simulink model "upperLimb"  (R2017b)
settings: Solver=VariableStepAuto  StartTime=0.0  StopTime=10.0  RelTol=1e-3
settings Model: Creator=user  LastModifiedBy=user

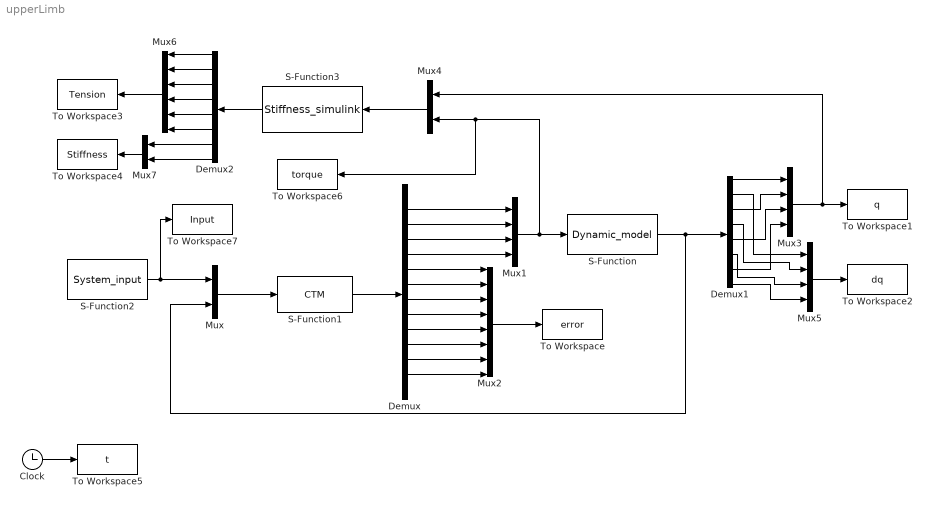
== system upperLimb ==
  Clock : Clock
  Demux : Demux  Outputs=12
  Demux1 : Demux  Outputs=8
  Demux2 : Demux  Outputs=8
  Mux : Mux  Inputs=2
  Mux1 : Mux
  Mux2 : Mux  Inputs=8
  Mux3 : Mux
  Mux4 : Mux  Inputs=2
  Mux5 : Mux
  Mux6 : Mux  Inputs=6
  Mux7 : Mux  Inputs=2
  S-Function : S-Function  FunctionName=Dynamic_model  SFunctionDeploymentMode=off  EnableBusSupport=off
  S-Function1 : S-Function  FunctionName=CTM  SFunctionDeploymentMode=off  EnableBusSupport=off
  S-Function2 : S-Function  FunctionName=System_input  SFunctionDeploymentMode=off  EnableBusSupport=off
  S-Function3 : S-Function  FunctionName=Stiffness_simulink  SFunctionDeploymentMode=off  EnableBusSupport=off
  To Workspace : ToWorkspace  VariableName=error  SaveFormat=Timeseries  SampleTime=-1
  To Workspace1 : ToWorkspace  VariableName=q  SaveFormat=Timeseries  SampleTime=-1
  To Workspace2 : ToWorkspace  VariableName=dq  SaveFormat=Timeseries  SampleTime=-1
  To Workspace3 : ToWorkspace  VariableName=Tension  SaveFormat=Timeseries  SampleTime=-1
  To Workspace4 : ToWorkspace  VariableName=Stiffness  SaveFormat=Timeseries  SampleTime=-1
  To Workspace5 : ToWorkspace  VariableName=t  SaveFormat=Timeseries  SampleTime=-1
  To Workspace6 : ToWorkspace  VariableName=torque  SaveFormat=Timeseries  SampleTime=-1
  To Workspace7 : ToWorkspace  VariableName=Input  SaveFormat=Timeseries  SampleTime=-1
  wires:
  S-Function2/1 -> To Workspace7/1, Mux/1
  Mux/1 -> S-Function1/1
  S-Function1/1 -> Demux/1
  Demux/1 -> Mux1/1
  Demux/2 -> Mux1/2
  Demux/3 -> Mux1/3
  Demux/4 -> Mux1/4
  Mux1/1 -> To Workspace6/1, Mux4/2, S-Function/1
  Demux/6 -> Mux2/2
  Demux/7 -> Mux2/3
  Demux/8 -> Mux2/4
  Demux/9 -> Mux2/5
  Demux/10 -> Mux2/6
  Demux/11 -> Mux2/7
  Demux/12 -> Mux2/8
  Demux/5 -> Mux2/1
  Mux2/1 -> To Workspace/1
  Mux3/1 -> Mux4/1, To Workspace1/1
  Mux4/1 -> S-Function3/1
  Mux5/1 -> To Workspace2/1
  S-Function/1 -> Mux/2, Demux1/1
  S-Function3/1 -> Demux2/1
  Mux6/1 -> To Workspace3/1
  Demux2/1 -> Mux6/1
  Demux2/2 -> Mux6/2
  Demux2/3 -> Mux6/3
  Demux2/4 -> Mux6/4
  Demux2/5 -> Mux6/5
  Demux2/6 -> Mux6/6
  Demux2/7 -> Mux7/1
  Demux2/8 -> Mux7/2
  Mux7/1 -> To Workspace4/1
  Demux1/1 -> Mux3/1
  Demux1/3 -> Mux3/2
  Demux1/5 -> Mux3/3
  Demux1/7 -> Mux3/4
  Demux1/2 -> Mux5/1
  Demux1/4 -> Mux5/2
  Demux1/6 -> Mux5/3
  Demux1/8 -> Mux5/4
  Clock/1 -> To Workspace5/1
